simulink model "model2"  (R2020b)
settings: Solver=VariableStepAuto  StartTime=0.0  StopTime=100  RelTol=1e-3
settings Model: PauseTimes=50  Creator=lulut  LastModifiedBy=lulut

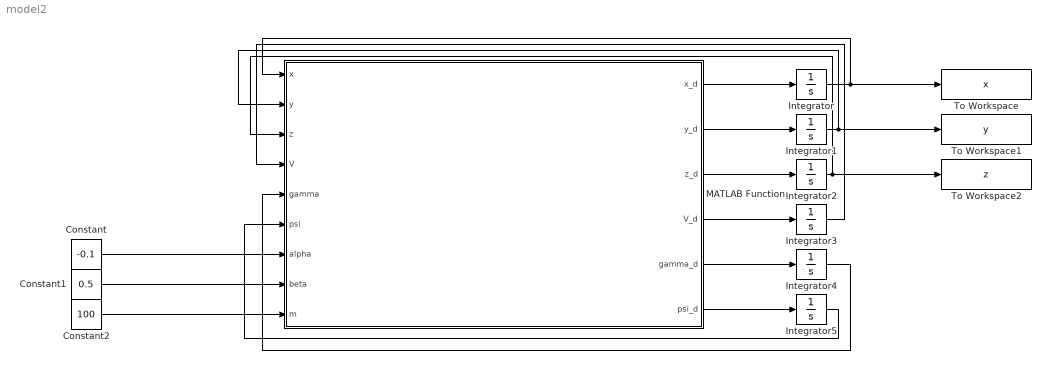
== system model2 ==
  Constant : Constant  Value=-0.1
  Constant1 : Constant  Value=0.5
  Constant2 : Constant  Value=100
  Integrator{,1,4..5} (4 alike) : Integrator
  Integrator2 : Integrator  InitialCondition=300
  Integrator3 : Integrator  InitialCondition=280
  MATLAB Function : MATLAB Function  TreatAsAtomicUnit=on
  To Workspace : ToWorkspace  VariableName=x  SampleTime=-1
  To Workspace1 : ToWorkspace  VariableName=y  SampleTime=-1
  To Workspace2 : ToWorkspace  VariableName=z  SampleTime=-1
  wires:
  MATLAB Function/1(x_d) -> Integrator/1
  MATLAB Function/2(y_d) -> Integrator1/1
  MATLAB Function/3(z_d) -> Integrator2/1
  MATLAB Function/4(V_d) -> Integrator3/1
  MATLAB Function/5(gamma_d) -> Integrator4/1
  MATLAB Function/6(psi_d) -> Integrator5/1
  Constant/1 -> MATLAB Function/7(alpha)
  Constant1/1 -> MATLAB Function/8(beta)
  Constant2/1 -> MATLAB Function/9(m)
  Integrator/1 -> To Workspace/1, MATLAB Function/1(x)
  Integrator1/1 -> To Workspace1/1, MATLAB Function/2(y)
  Integrator2/1 -> To Workspace2/1, MATLAB Function/3(z)
  Integrator3/1 -> MATLAB Function/4(V)
  Integrator4/1 -> MATLAB Function/5(gamma)
  Integrator5/1 -> MATLAB Function/6(psi)

== matlab function model2/MATLAB Function ==
  data: x_d output double size=1; x input double size=1; y input double size=1; z input double size=1; V input double size=1; gamma input double size=1; psi input double size=1; alpha input double size=1; beta input double size=1; m input double size=1; y_d output double size=1; z_d output double size=1; V_d output double size=1; gamma_d output double size=1; psi_d output double size=1
function [x_d,y_d,z_d,V_d,gamma_d,psi_d] = model_2(x ,y ,z ,V ,gamma, psi,alpha,beta,m)

%这是进一步考虑飞行器气动特性的平面大地三维质点动力学模型；
%攻角和侧滑角：alpha 和 beta 为主要输入；
%status = [x y z V gamma psi]；
%
S_ref = 0.48; %飞行器特征面积
%C_d = 0.25; %飞行器阻力系数
g = 9.8061;  %平面大地假设下的重力加速度
rou_0 = 1.225; %海平面空气密度
H = 7200;  %大气密度计算常值

rou = rou_0 * exp(-z/H);

C_d = 0.000508 * (alpha^2 + beta^2) + 0.004228 * (alpha^2 + beta^2)^(1/2) + 0.0161;
C_l = 0.04675 * alpha - 0.10568;
C_n = 0.04675 * beta - 0.10568;

D = 0.5 * rou * V^2 * S_ref * C_d;
L = 0.5 * rou * V^2 * S_ref * C_l;
N = 0.5 * rou * V^2 * S_ref * C_n; 

x_d = V * cos(gamma) * sin(psi);
y_d = V * cos(gamma) * cos(psi);
z_d = V * sin(gamma);
V_d = -D/m - g*sin(gamma);
gamma_d = L/(m*V) - g* cos(gamma)/V;
psi_d = N/(m*V*cos(gamma));
